simulink model "PowerTrain_Simulink_ModelValidation"  (R2021a)
settings: Solver=ode23tb  StartTime=0.0  StopTime=796.8349  RelTol=1e-3
undefined symbols (not defined in the file): QuadrotorPowerTrainModel_Object
settings Model: OrderedModelArguments=off  Creator=renkert2  LastModifiedBy=renkert2
settings SolverCC: AlgebraicLoopSolver=TrustRegion
settings DebuggingCC: SFMachineParentedDataDiag=warning

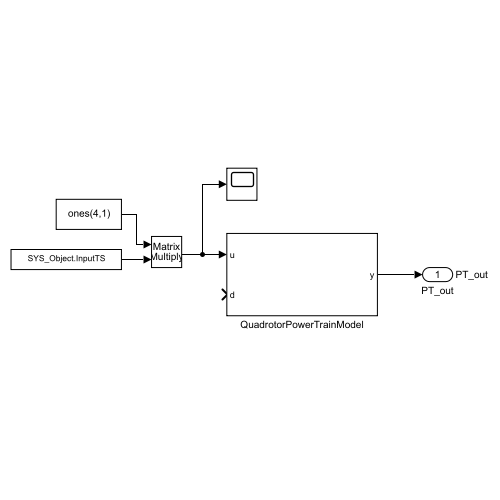
[thumbnail: Simulink's stored preview of the top-level diagram]
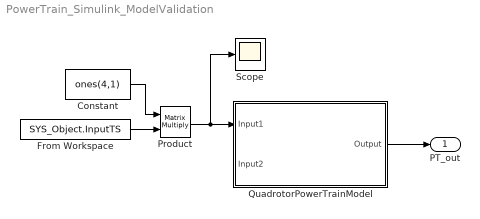
== system PowerTrain_Simulink_ModelValidation ==
  Constant : Constant  Value=ones(4,1)
  From Workspace : FromWorkspace  VariableName=SYS_Object.InputTS
  Product : Product  Multiplication=Matrix(*)
  QuadrotorPowerTrainModel : Subsystem  mask{x_0=QuadrotorPowerTrainModel_Object.x0}
  Scope : Scope
  PT_out : Outport  SignalName=PT_out
  wires:
  QuadrotorPowerTrainModel/1(Output) -> PT_out/1
  Constant/1 -> Product/1
  Product/1 -> QuadrotorPowerTrainModel/1(Input1), Scope/1
  From Workspace/1 -> Product/2

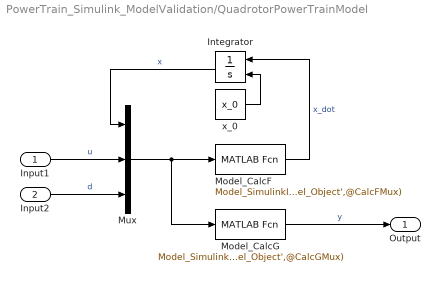
== system PowerTrain_Simulink_ModelValidation/QuadrotorPowerTrainModel ==
  Input1 : Inport  PortDimensions=[QuadrotorPowerTrainModel_Object.Nu,1]
  Input2 : Inport  Port=2  PortDimensions=[QuadrotorPowerTrainModel_Object.Nd,1]
  Integrator : Integrator  InitialConditionSource=external
  Model_CalcF : MATLABFcn  MATLABFcn=Model_SimulinkInterpretedFunction(u,'PowerTrain_Simulink_ModelValidation','QuadrotorPowerTrainModel_Object',@CalcFMux)  OutputDimensions=QuadrotorPowerTrainModel_Object.Nx
  Model_CalcG : MATLABFcn  MATLABFcn=Model_SimulinkInterpretedFunction(u,'PowerTrain_Simulink_ModelValidation','QuadrotorPowerTrainModel_Object',@CalcGMux)  OutputDimensions=QuadrotorPowerTrainModel_Object.Ny
  Mux : Mux  Inputs=3
  x_0 : Constant  Value=x_0  VectorParams1D=off
  Output : Outport
  wires:
  Mux/1 -> Model_CalcF/1, Model_CalcG/1
  Integrator/1 -> Mux/1  "x"
  Input2/1 -> Mux/3  "d"
  x_0/1 -> Integrator/2
  Model_CalcG/1 -> Output/1  "y"
  Input1/1 -> Mux/2  "u"
  Model_CalcF/1 -> Integrator/1  "x_dot"
